simulink model "conv_rect_pulse"  (R2016a)
settings: Solver=VariableStepAuto  StartTime=0.0  StopTime=10.0  RelTol=1e-3
libraries: dspsrcs4 x2, dspsigops x1
settings Model: Creator=Chris  LastModifiedBy=Chris

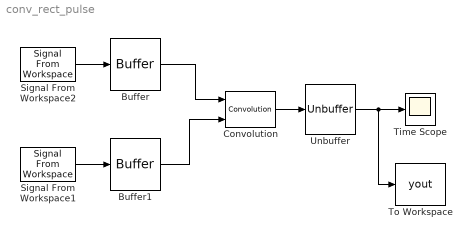
== system conv_rect_pulse ==
  Buffer : Buffer  N=16  TreatMby1Signals=One channel
  Buffer1 : Buffer  N=16  TreatMby1Signals=One channel
  Convolution : dspsigops/Convolution  domain=Time  outputDataTypeStr=Inherit: Same as accumulator  outputLastDataTypeStr=Inherit: Same as accumulator  outputMin=[]  outputMax=[]  roundingMode=Floor  overflowMode=off
  Signal From Workspace1 : dspsrcs4/Signal From Workspace  X=[1 1 1 1]  Ts=1  nsamps=1  OutputAfterFinalValue=Setting to zero  ignoreOrWarnInputAndFrameLengths=off  OutputFrames=on
  Signal From Workspace2 : dspsrcs4/Signal From Workspace  X=[1 1 1]  Ts=1  nsamps=1  OutputAfterFinalValue=Setting to zero  ignoreOrWarnInputAndFrameLengths=off  OutputFrames=on
  Time Scope : Scope
  To Workspace : ToWorkspace  VariableName=yout  SampleTime=-1
      settings: Save2DSignal=2-D array (concatenate along first dimension)
  Unbuffer : Unbuffer  SampleBasedProcessing=Same as frame based
  wires:
  Signal From Workspace1/1 -> Buffer1/1
  Buffer1/1 -> Convolution/2
  Convolution/1 -> Unbuffer/1
  Unbuffer/1 -> Time Scope/1, To Workspace/1
  Buffer/1 -> Convolution/1
  Signal From Workspace2/1 -> Buffer/1
